simulink model "doc_moqpskmod_sb"  (R2014a)
settings: Solver=FixedStepDiscrete  StartTime=0.0  StopTime=10.0  RelTol=1e-3
libraries: commdigbbndpm3 x2, commutil2 x1
settings Model: Creator=The MathWorks Inc.
settings DataIOCC: SignalLoggingSaveFormat=ModelDataLogs
settings OptimizationCC: BlockReduction=off  ExpressionDepthLimit=2147483647  EfficientMapNaN2IntZero=off
settings DebuggingCC: UnderspecifiedInitializationDetection=Classic  FcnCallInpInsideContextMsg=UseLocalSettings  StateNameClashWarn=warning  StrictBusMsg=Warning
settings GRTTargetCC: CombineOutputUpdateFcns=off  GRTInterface=on

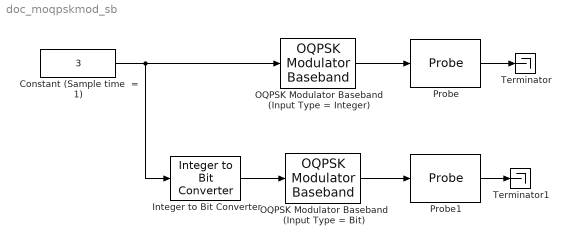
== system doc_moqpskmod_sb ==
  Constant (Sample time  = 1) : Constant  Value=3  VectorParams1D=off  SampleTime=1  FramePeriod=6
  Integer to Bit Converter : commutil2/Integer to Bit Converter  nbits=2  signedInputValues=Unsigned  bitOrder=MSB first  outDtype=double
  OQPSK Modulator Baseband (Input Type = Bit) : commdigbbndpm3/OQPSK Modulator Baseband  InType=Bit  Ph=0  RateOptions=Allow multirate processing  outDtype=double  outWordLen=16  outUDDataType=sfix(16)  outFracLenMode=Best precision  outFracLen=15
  OQPSK Modulator Baseband (Input Type = Integer) : commdigbbndpm3/OQPSK Modulator Baseband  InType=Integer  Ph=0  RateOptions=Allow multirate processing  outDtype=double  outWordLen=16  outUDDataType=sfix(16)  outFracLenMode=Best precision  outFracLen=15
  Probe : Probe  ProbeWidth=off  ProbeComplexSignal=off
  Probe1 : Probe  ProbeWidth=off  ProbeComplexSignal=off
  Terminator : Terminator
  Terminator1 : Terminator
  wires:
  Constant (Sample time  = 1)/1 -> OQPSK Modulator Baseband (Input Type = Integer)/1, Integer to Bit Converter/1
  OQPSK Modulator Baseband (Input Type = Integer)/1 -> Probe/1
  OQPSK Modulator Baseband (Input Type = Bit)/1 -> Probe1/1
  Probe/1 -> Terminator/1
  Probe1/1 -> Terminator1/1
  Integer to Bit Converter/1 -> OQPSK Modulator Baseband (Input Type = Bit)/1
